simulink model "EPT"  (R2019b)
settings: Solver=FixedStepDiscrete  StartTime=0.0  StopTime=5  FixedStep=0.005  RelTol=1e-3  EnableMultiTasking=on
PreLoadFcn:
  | try, model_open; catch, disp('Error occurred while executing model pre-load callback: model_open.m'); disp('Please assure that the MATLAB working directory is set to the model directory before opening.'); end
InitFcn:
  | try, model_open; catch, end
undefined symbols (not defined in the file or in its folder): Bridge, GCM, H, ln, raptor_get_param_eval, raptor_get_safe_string, raptor_xcp_function
libraries: Raptor_lib x2810, simulink x374, hdlsllib x19
(part 45 of 45)

== matlab function EPT/Foreground_TimeBase_5ms/CAN/CAN2_exec/Remote DA /Remote DA Status G22 (ESS-OBU#3)/Vcell Min//Max/Sort ==
  data: array input; Max output; Min output; Max_order output; Min_order output
function [Max,Min,Max_order,Min_order] = fcn(array)
[u1, u2]  = sort(array, 'descend');
length(array);
Max=u1(1);
Min=u1(length(array));
Max_order=u2(1);
Min_order=u2(length(array));
